simulink model "Lab1_1_sol"  (R2025a)
settings: Solver=ode45  StartTime=0.0  StopTime=10000/20e6  RelTol=1e-3  EnableMultiTasking=on
undefined symbols (not defined in the file): fdesignblkfcn, gcbh, xc7vx485tffg1157, xlfda_numerator
libraries: hdlBasic x3, dspfdesign x1, hdlUtilities x1, vmcUtilities x1
settings Model: Creator=danielm  LastModifiedBy=robg
settings SolverCC: AlgebraicLoopSolver=TrustRegion
settings DataIOCC: LimitDataPoints=on  SaveFormat=Array  ReturnWorkspaceOutputs=off
settings OptimizationCC: LifeSpan=inf
settings DebuggingCC: UnderspecifiedInitializationDetection=Classic  MergeDetectMultiDrivingBlocksExec=none  SolverPrmCheckMsg=warning  UnconnectedInputMsg=warning  UnconnectedOutputMsg=warning  UnconnectedLineMsg=warning  SFUnexpectedBacktrackingDiag=warning  SFNoUnconditionalDefaultTransitionDiag=warning  SFExecutionAtInitializationDiag=none  ArithmeticOperatorsInVariantConditions=warning
settings HardwareCC: ProdBitPerPointer=32.0  ProdBitPerSizeT=32.0  ProdBitPerPtrDiffT=32.0  ProdLargestAtomicFloat=None  ProdIntDivRoundTo=Undefined  ProdEndianess=Unspecified  ProdWordSize=32.0  ProdHWDeviceType=32-bit Generic
settings ModelReferenceCC: EnableRefExpFcnMdlSchedulingChecks=on  PropagateSignalLabelsOutOfModel=off
settings SFSimCC: SimUseLocalCustomCode=off  CustomCodeUndefinedFunction=UseInterfaceOnly
settings RTWCC: RTWUseLocalCustomCode=off  GPUComputeCapability=3.5  DLArmComputeVersion=19.05
settings CodeAppCC: StateflowObjectComments=on
settings GRTTargetCC: TargetLangStandard=C89/C90 (ANSI)
settings ConfigComp: CovMetricSettings=dw  CovSaveCumulativeToWorkspaceVar=on  CovSaveSingleToWorkspaceVar=on  CovExternalEMLEnable=off  CovSFcnEnable=off

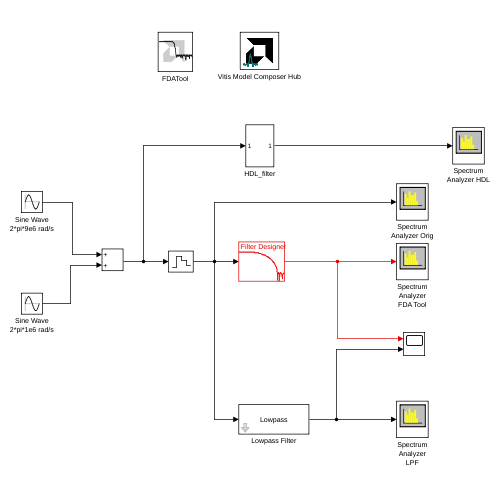
[thumbnail: Simulink's stored preview of the top-level diagram]
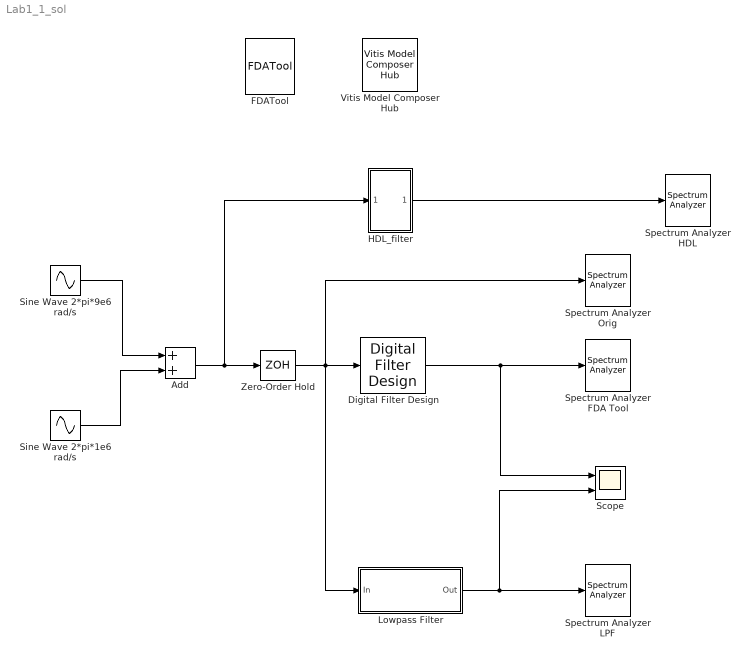
== system Lab1_1_sol ==
  Add : Sum
  Digital Filter Design : dspfdesign/Digital Filter Design  mwdsp_browser_bugfix_var=off
  FDATool : hdlUtilities/FDATool  block_type=fdatool
      settings: infoedit=FDATool
  HDL_filter : Subsystem
  Lowpass Filter : Subsystem  DialogController=fdesignblkfcn  InitFcn=fdesignblkfcn(gcbh, {'InitFcn'});  mask(Lowpass Filter){}
      mask help: Design a lowpass filter
      settings: CopyFcn=fdesignblkfcn(gcbh, {'CopyFcn'});
      mask Help: helpview(mapfilelocation('dsp'), 'dsplowpassfilter');
      mask Display: disp('Lowpass')
  Scope : Scope  NumInputPorts=2
      settings: ActiveDisplayYMinimum=-5  ActiveDisplayYMaximum=5
  Sine Wave 2*pi*1e6 rad/s : Sin  Frequency=2*pi*1e6  SampleTime=0
  Sine Wave 2*pi*9e6 rad/s : Sin  Frequency=2*pi*9e6  SampleTime=0
  Spectrum Analyzer FDA Tool : SpectrumAnalyzer  WindowPosition=[833 109 560 420]  Visible=on  Method=Welch  SampleRate=20000000  AveragingMethod=Exponential  YLimits=[-187.0838,47.1991]  ChannelNames="[\"\"]"  AllowFFTLengthLessThanSamplesPerUpdate=on  DefaultConfigurationName=spbscopes.SpectrumAnalyzerBlockCfg
  Spectrum Analyzer LPF : SpectrumAnalyzer  WindowPosition=[1026 106 568 420]  Visible=on  Method=Welch  SampleRate=20000000  AveragingMethod=Exponential  YLimits=[-187.1897,47.1957]  ChannelNames="[\"\"]"  AllowFFTLengthLessThanSamplesPerUpdate=on  DefaultConfigurationName=spbscopes.SpectrumAnalyzerBlockCfg
  Spectrum Analyzer HDL : SpectrumAnalyzer  WindowPosition=[241 103 568 420]  Visible=on  Method=Welch  SampleRate=20000000  AveragingMethod=Exponential  YLimits=[-207.5529,49.4734]  ChannelNames="[\"\"]"  AllowFFTLengthLessThanSamplesPerUpdate=on  DefaultConfigurationName=spbscopes.SpectrumAnalyzerBlockCfg
  Spectrum Analyzer Orig : SpectrumAnalyzer  WindowPosition=[241 103 568 420]  Visible=on  Method=Welch  SampleRate=20000000  AveragingMethod=Exponential  YLimits=[-153.2838,43.4257]  ChannelNames="[\"\"]"  AllowFFTLengthLessThanSamplesPerUpdate=on  DefaultConfigurationName=spbscopes.SpectrumAnalyzerBlockCfg
  Vitis Model Composer Hub : vmcUtilities/Vitis Model Composer Hub  Tag=genX  CodeGeneration=off  StartColumn=1  NumberOfColumns=1  TargetDirectory=./code  exportDesign=off  analyzeDesign=off  validateDesignOnHw=off  ExportType=AI Engines  IpVendor=xilinx.com  IpLibrary=hls  IpVersion=1.0  IpHWLanguage=Verilog  AieCompilerOptions={}  AieSimulatorOptions={}  CreateTestbench=off  TestbenchStackSize=10  RunRtlSim=off  RunCSim=off  RunAieSim=off  enableSimulationTimeout=on  enableGraphIterations=on  AieSimTimeout=50000  AieGraphIterations=-1  RunAieSimProfiling=off  LaunchVitisAnalyzer=off  PlotOutput=off  RunX86Sim=off  X86SimTimeout=10  GenHwImage=off  GenLibadfXo=off  GenHwValidationCode=off  PlatformType=Not Specified  HwSystemType=Baremetal  HwValidationTarget=hw  ProjDevice=xc7vx485tffg1157-3  ProjDevicePart=xc7vx485tffg1157-3  SamplePeriod=-1  ClockFrequency=200  DataPathParallelism=1  xilinxfamily=virtex7  part=xc7vx485t  speed=-3  package=ffg1157  directory=./netlist  testbench=off  incr_netlist=off  synthesis_tool=Vivado  clock_wrapper=Clock Enables  dbl_ovrd=According to Block Masks  dcm_input_clock_period=10  sysclk_period=50  simulink_period=1/20e6  eval_field=0  IPInfoJsonString="{\"HDLSubsystem\":{\"SubsystemName\":\"HDL_filter\",\"IPName\":\"HDL_filter\",\"IPLibrary\":\"VMC\",\"IPVendor\":\"User Company\",\"IPVersion\":\"1.0\"}}"  LogFileName=''  NThreads=4
  Zero-Order Hold : ZeroOrderHold  SampleTime=1/20e6
  wires:
  Sine Wave 2*pi*9e6 rad/s/1 -> Add/1
  Sine Wave 2*pi*1e6 rad/s/1 -> Add/2
  Digital Filter Design/1 -> Scope/1, Spectrum Analyzer FDA Tool/1
  Zero-Order Hold/1 -> Spectrum Analyzer Orig/1, Lowpass Filter/1(In), Digital Filter Design/1
  Lowpass Filter/1(Out) -> Scope/2, Spectrum Analyzer LPF/1
  Add/1 -> HDL_filter/1(In1), Zero-Order Hold/1
  HDL_filter/1(Out1) -> Spectrum Analyzer HDL/1

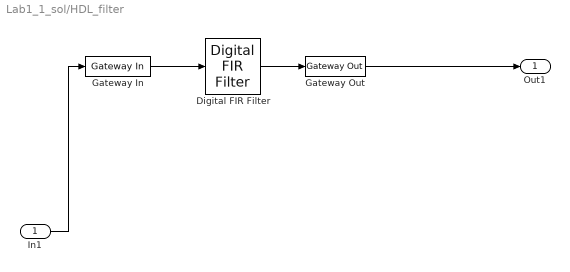
== system Lab1_1_sol/HDL_filter ==
  In1 : Inport
  Digital FIR Filter : hdlBasic/Digital FIR Filter  coeff_source=off  coefficientvector=xlfda_numerator([bdroot, '/FDATool'])  coeff_calulate=on  coefficient_width=19  coefficient_fractional_bits=19  interpolation_filter_rate=1  decimation_filter_rate=1  fda_coefficientvector=[-0.0024 -0.0042 0.0095 0.0200 -0.0380 -0.0696 0.1374 0.4472 0.4472 0.1374 -0.0696 -0.0380 0.0200 0.0095 -0.0042 -0.0024]  simulation_type=fast_sim  simulation_model=sysgen:fir_macro  XmcBlockStatus=1  maskContainerNames=group1  block_type=fir_macro  block_config=sysgen:fir_macro_config
  Gateway In : hdlBasic/Gateway In  gui_display_data_type=Fixed-point  arith_type=Signed (2's comp)  n_bits=16  bin_pt=14  preci_type=Single  exp_width=8  frac_width=24  rows=1  columns=1  quantization="Round  (unbiased: +/- Inf)"  overflow=Saturate  period=1/20e6  UseAsADC=off  ADCChannel='1'  interface=None  automatic_assignment=on  address_offset=hex2dec('00')  intf_name=''  intf_description=''  default_value=0  timing_constraint=None  locs_specified=off  LOCs={}  io_standard={}  inherit_from_input=off  hdl_port=on  XmcBlockStatus=1  maskContainerNames=group4  block_type=gatewayin  block_config=sysgen:gateway_in_config  block_width_w=590  block_height_w=620  block_width=640  block_height=850
  Gateway Out : hdlBasic/Gateway Out  inherit_from_input=off  bool_to_boolean=off  hdl_port=on  rows=1  columns=1  UseAsDAC=off  DACChannel='1'  interface=None  automatic_assignment=on  address_offset=hex2dec('00')  intf_name=''  intf_description=''  timing_constraint=None  locs_specified=off  LOCs={}  io_standard={}  XmcBlockStatus=1  maskContainerNames=group4  block_type=gatewayout  block_config=sysgen:gateway_out_config  block_width_w=590  block_height_w=620  block_width=620  block_height=750
  Out1 : Outport
  wires:
  Gateway In/1 -> Digital FIR Filter/1
  Digital FIR Filter/1 -> Gateway Out/1
  In1/1 -> Gateway In/1
  Gateway Out/1 -> Out1/1

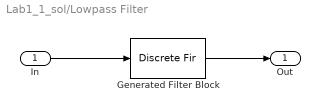
== system Lab1_1_sol/Lowpass Filter ==
  In : Inport
  Generated Filter Block : DiscreteFir  Tag=BlockMethodSubSystem  Coefficients=[0.006802019168867246 -0.0018271019166862348 -0.051845131678638426 0.0057350837125695478 0.29497742250115677 0.49199741364352395 0.29497742250115677 0.0057350837125695478 -0.051845131678638426 -0.0018271019166862348 0.006802019168867246]  InputProcessing=Columns as channels (frame based)
  Out : Outport  VectorParamsAs1DForOutWhenUnconnected=off
  wires:
  In/1 -> Generated Filter Block/1
  Generated Filter Block/1 -> Out/1
